simulink subsystem "MPC10_nlpsol"  (R2022b)
settings: Solver=VariableStepAuto  StartTime=0.0  StopTime=10.0  RelTol=1e-3
undefined symbols (not defined in the file): param_global, param_jointspace_ct, param_MPC10, param_robot, param_weight_init
settings Model: Creator=emu  LastModifiedBy=emu
settings OptimizationCC: ReuseModelBlockBuffer=on

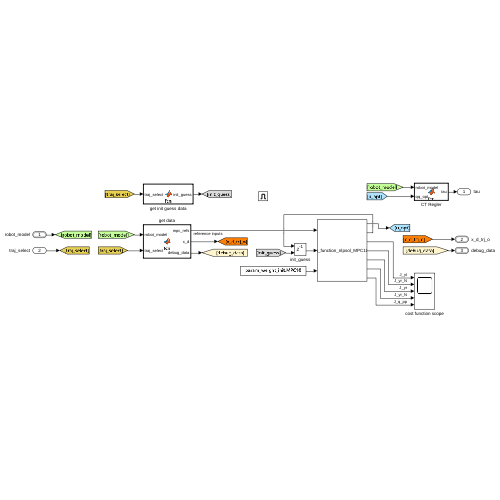
[thumbnail: Simulink's stored preview of the top-level diagram]
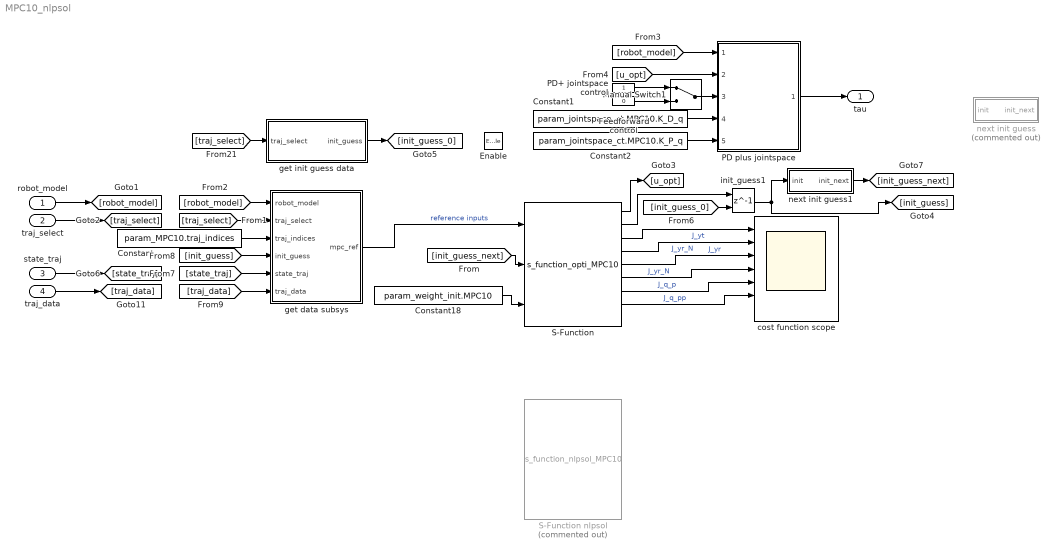
== system MPC10_nlpsol ==
  robot_model : Inport  OutDataTypeStr=Bus: robot_model
  traj_select : Inport  Port=2
  state_traj : Inport  Port=3  OutDataTypeStr=Bus: state_traj_bus
  traj_data : Inport  Port=4  OutDataTypeStr=Bus: traj_data_bus
  Enable : EnablePort
  Constant : Constant  Value=param_MPC10.traj_indices
  Constant1 : Constant  Value=param_jointspace_ct.MPC10.K_D_q
  Constant18 : Constant  Value=param_weight_init.MPC10  VectorParams1D=off
  Constant2 : Constant  Value=param_jointspace_ct.MPC10.K_P_q
  Feedforward control : Constant  Value=0
  Manual Switch1 : ManualSwitch
  PD plus jointspace : Subsystem  ReferencedSubsystem=closed_loop_kin_mpc_pdplus_control_refsys
  PD+ jointspace control : Constant
  S-Function : S-Function  FunctionName=s_function_opti_MPC10  SFunctionModules='MPC10'  SFunctionDeploymentMode=off  EnableBusSupport=off
  S-Function nlpsol : S-Function  Commented=on  FunctionName=s_function_nlpsol_MPC10  Parameters='s_functions/fr3_no_hand_6dof/MPC10.casadi', 'MPC10'  SFunctionModules='MPC10'  SFunctionDeploymentMode=off  EnableBusSupport=off
  cost function scope : Scope  NumInputPorts=7
  get data subsys : Subsystem
  get init guess data : MATLAB Function  TreatAsAtomicUnit=on
  init_guess1 : Delay  DelayLength=1  InitialConditionSource=Input port  InitialCondition=1  SampleTime=param_global.Ta
      settings: InputPortMap=u0,p4
  next init guess : MATLAB Function  Commented=on  TreatAsAtomicUnit=on
  next init guess1 : MATLAB Function  TreatAsAtomicUnit=on
  tau : Outport
  wires:
  Constant2/1 -> PD plus jointspace/5
  Constant1/1 -> PD plus jointspace/4
  Manual Switch1/1 -> PD plus jointspace/3
  [robot_model] -> PD plus jointspace/1
  [u_opt] -> PD plus jointspace/2
  Feedforward control/1 -> Manual Switch1/2
  PD plus jointspace/1 -> tau/1
  PD+ jointspace control/1 -> Manual Switch1/1
  [traj_data] -> get data subsys/6(traj_data)
  traj_data/1 -> [traj_data]
  [init_guess] -> get data subsys/4(init_guess)
  [init_guess_0] -> init_guess1/2
  S-Function/2 -> init_guess1/1
  init_guess1/1 -> next init guess1/1(init), [init_guess]
  get data subsys/1(mpc_ref) -> S-Function/1  "reference inputs"
  Constant/1 -> get data subsys/3(traj_indices)
  [robot_model] -> get data subsys/1(robot_model)
  [traj_select] -> get data subsys/2(traj_select)
  S-Function/1 -> [u_opt]
  S-Function/5 -> cost function scope/3  "J_yr"
  S-Function/3 -> cost function scope/1  "J_yt"
  Constant18/1 -> S-Function/3
  get init guess data/1(init_guess) -> [init_guess_0]
  robot_model/1 -> [robot_model]
  S-Function/4 -> cost function scope/2  "J_yr_N"
  traj_select/1 -> [traj_select]
  S-Function/6 -> cost function scope/4  "J_yr_N"
  [traj_select] -> get init guess data/1(traj_select)
  S-Function/7 -> cost function scope/5  "J_q_p"
  state_traj/1 -> [state_traj]
  [state_traj] -> get data subsys/5(state_traj)
  next init guess1/1(init_next) -> [init_guess_next]
  [init_guess_next] -> S-Function/2
  S-Function/8 -> cost function scope/6  "J_q_pp"

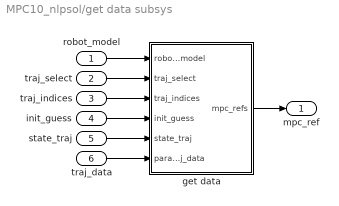
== system MPC10_nlpsol/get data subsys ==
  robot_model : Inport  OutDataTypeStr=Bus: robot_model
  traj_select : Inport  Port=2
  traj_indices : Inport  Port=3
  init_guess : Inport  Port=4
  state_traj : Inport  Port=5  OutDataTypeStr=Bus: state_traj_bus
  traj_data : Inport  Port=6  OutDataTypeStr=Bus: traj_data_bus
  get data : MATLAB Function  TreatAsAtomicUnit=on
  mpc_ref : Outport
  wires:
  state_traj/1 -> get data/5(state_traj)
  robot_model/1 -> get data/1(robot_model)
  traj_select/1 -> get data/2(traj_select)
  traj_indices/1 -> get data/3(traj_indices)
  get data/1(mpc_refs) -> mpc_ref/1
  init_guess/1 -> get data/4(init_guess)
  traj_data/1 -> get data/6(param_traj_data)

== matlab function MPC10_nlpsol/get data subsys/get data ==
  settings: updateMethod=DISCRETE  sampleTime=param_global.Ta
  data: mpc_refs output; robot_model input Bus: robot_model; traj_select input; traj_indices input; init_guess input; state_traj input Bus: state_traj_bus; param_robot parameter; param_traj_data input
function mpc_refs  = fcn(robot_model, traj_select, traj_indices, init_guess, state_traj, param_robot, param_traj_data)
persistent cnt;
persistent run_flag;

if(isempty(cnt))
    cnt = 1;
    run_flag = 0;
end

n_red = param_robot.n_red;
n_indices = param_robot.n_indices;

traj_indices = traj_indices + (cnt-1);
N_MPC = length(traj_indices)-1;

% Parameters
q    = robot_model.q;      % generalized coordinates
q_p  = robot_model.q_p;  % time derivative of generalized coordinates

x_k = [q(n_indices);q_p(n_indices)];

% Assemble vector of recieved output measurements
p_d     = param_traj_data.p_d(   1:3, traj_indices, traj_select);
q_d     = param_traj_data.q_d(   1:4, traj_indices, traj_select);

y_d = [p_d; q_d];

%% Reference out
N_u = n_red*1;
N_q = n_red * (N_MPC+1);
q_k_prev = init_guess(1+N_u : N_u+N_q);
mpc_refs = [x_k(:); y_d(:); q_k_prev(:)]';


[run_flag, cnt] = update_traj_cnt(state_traj, run_flag, cnt, param_traj_data.N);

== matlab function MPC10_nlpsol/get init guess data ==
  data: traj_select input; param_MPC10_init_guess parameter; init_guess output
function init_guess   = fcn(traj_select, param_MPC10_init_guess)

init_guess = param_MPC10_init_guess.init_guess(traj_select,:);

== matlab function MPC10_nlpsol/next init guess1 ==
  data: init input; init_next output; param_MPC10 parameter; param_robot parameter; param_global parameter
function init_next = fcn(init, param_MPC10, param_robot, param_global)
param_MPC = param_MPC10;

Ta = param_global.Ta;
dt_arr = param_MPC.int_times;
N_MPC = param_MPC.N;
n_red = param_robot.n_red;
N_u =    n_red * N_MPC;
N_x = (2*n_red)*(N_MPC+1);
%N_q = (  n_red)*(N_MPC+1);

N = 0;

init_next = init';

%% u next
u_idx = N + [1:N_u];       N = N + length(u_idx);
u_idx_2d = reshape(u_idx, n_red, (N_MPC));
u_idx_2d(:, 1:end-1) = u_idx_2d(:, 2:end);
u_init = init(u_idx_2d);

du = (u_init(:, 2:end) - u_init(:, 1:end-1))./dt_arr(1:end-1);
u_next = u_init(:, 1:end-1) + du * Ta;

u_idx_m1 = u_idx_2d(:, 1:end-1);
init_next(u_idx_m1) = u_next;
%% x next
x_idx = N + [1:N_x];       N = N + length(x_idx);
x_idx_2d = reshape(x_idx, 2*n_red, (N_MPC+1));
x_idx_2d(:, 1:end-1) = x_idx_2d(:, 2:end);
x_init = init(x_idx_2d);

dx = (x_init(:, 2:end) - x_init(:, 1:end-1))./dt_arr;
x_next = x_init(:, 1:end-1) + dx * Ta;

x_idx_m1 = x_idx_2d(:, 1:end-1);
init_next(x_idx_m1) = x_next;

== matlab function MPC10_nlpsol/next init guess ==
  data: init input; init_next output; param_MPC10 parameter; param_robot parameter; param_global parameter
function init_next = fcn(init, param_MPC10, param_robot, param_global)
param_MPC = param_MPC10;

Ta = param_global.Ta;
dt_arr = param_MPC.int_times;
N_MPC = param_MPC.N;
n_red = param_robot.n_red;
N_u = n_red * 1;
N_q = (n_red)*(N_MPC+1);

N = 0;

u_idx = N + [1:N_u];       N = N + length(u_idx);
q_idx = N + [1:N_q];       N = N + length(q_idx);
q_idx_2d = reshape(q_idx, n_red, (N_MPC+1));
q_idx_2d(:, 1:end-1) = q_idx_2d(:, 2:end);

q_init = init(q_idx_2d);

dq = (q_init(:, 2:end) - q_init(:, 1:end-1))./dt_arr;
q_next = q_init(:, 1:end-1) + dq * Ta;

x_idx_m1 = q_idx_2d(:, 1:end-1);

init_next = init';
init_next(x_idx_m1) = q_next;
